simulink model "DKSTDD_Bo_KDXCS_dieu_khien_DC_1c"  (R2019a)
settings: Solver=VariableStepAuto  StartTime=0.0  StopTime=5  RelTol=1e-3
libraries: powerlib x8
settings Model: Creator=Admin  LastModifiedBy=Admin

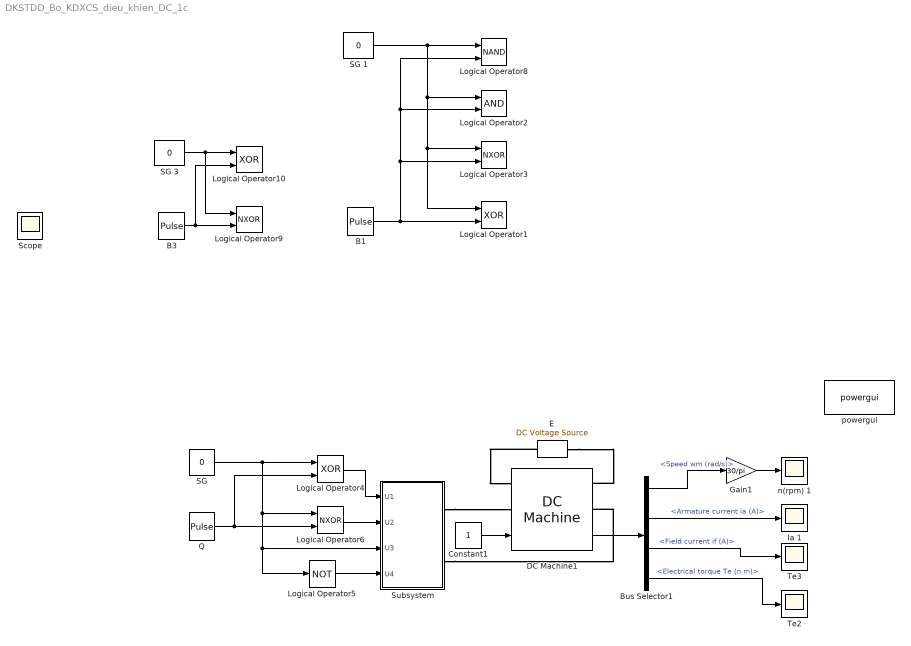
== system DKSTDD_Bo_KDXCS_dieu_khien_DC_1c ==
  B1 : DiscretePulseGenerator  PulseType=Time based  Period=0.002  PulseWidth=20
  B3 : DiscretePulseGenerator  PulseType=Time based  Period=0.002  PulseWidth=20
  Bus Selector1 : BusSelector  OutputSignals=Speed wm (rad/s),Armature current ia (A),Field current if (A),Electrical torque Te (n m)
  Constant1 : Constant
  DC Machine1 : powerlib/Machines/DC Machine  PresetModel=01: 5HP 240V 1750RPM Field:300V  MechanicalLoad=Torque TL  FieldType=Wound  ShowDetailedParameters=on  MeasurementBus=off  RLa=[2.581 0.028]  RLf=[281.3 156]  Laf=0.9483  MachineConstant=Torque constant (N.m/A)  Ke=1.8  Kt=1.8  J=0.02215  Bm=0.002953  Tf=0.5161  w0=1  Ifinit=1  TsPowergui=0  TsBlock=-1
  E : powerlib/Electrical Sources/DC Voltage Source  Amplitude=300  Measurements=None
  Gain1 : Gain  Gain=30/pi
  Ia 1 : Scope
  Logical Operator1 : Logic  Operator=XOR  AllPortsSameDT=off  OutDataTypeStr=boolean
  Logical Operator10 : Logic  Operator=XOR  AllPortsSameDT=off  OutDataTypeStr=boolean
  Logical Operator2 : Logic  AllPortsSameDT=off  OutDataTypeStr=boolean
  Logical Operator3 : Logic  Operator=NXOR  AllPortsSameDT=off  OutDataTypeStr=boolean
  Logical Operator4 : Logic  Operator=XOR  AllPortsSameDT=off  OutDataTypeStr=boolean
  Logical Operator5 : Logic  Operator=NOT  AllPortsSameDT=off  OutDataTypeStr=boolean
  Logical Operator6 : Logic  Operator=NXOR  AllPortsSameDT=off  OutDataTypeStr=boolean
  Logical Operator8 : Logic  Operator=NAND  AllPortsSameDT=off  OutDataTypeStr=boolean
  Logical Operator9 : Logic  Operator=NXOR  AllPortsSameDT=off  OutDataTypeStr=boolean
  Q : DiscretePulseGenerator  PulseType=Time based  Period=0.002  PulseWidth=20
  SG : Constant  Value=0
  SG 1 : Constant  Value=0
  SG 3 : Constant  Value=0
  Scope : Scope  NumInputPorts=4
  Subsystem : Subsystem
  Te2 : Scope
  Te3 : Scope
  n(rpm) 1 : Scope
  powergui : powerlib/powergui  Priority=1  SimulationMode=Continuous  SampleTime=50e-6  frequency=60  Iterations=50  frequencyindice=0  Pbase=100e6  ErrMax=1e-4  UnitsV=kV  UnitsW=MW  buscounter=0  FunctionMessages=off  echomessages=off  EnableUseOfTLC=off  CurrentSourceSwitches=off  DisableSnubberDevices=off  DisableRonSwitches=off  DisableVfSwitches=off  DisplayEquations=off  AutomaticDiscreteSolvers=off  SolverType=Tustin/Backward Euler (TBE)  Interpol=off  ExternalGateDelay=off  methode=off  Ts=100  x0status=blocks  SPID=on  SwTol=0  HookPort=off  NonlinearTolerance=0  nMaxIteration=15  ContinueOnMaxIteration=off  RestoreLinks=warning  ResistiveCurrentMeasurement=off  Frange=[0:2:500]  Ylog=off  Xlog=on  ShowGrid=off  save=off  variable=ZData  structure=0  ZoomFFT=off  StartTime=0.0  cycles=1  DisplayStyle=1  fundamental=60  FreqAxis=off  MaxFrequency=1000  frequencyindicesteady=1  RmsSteady=1  display=off
      settings: SourceProductName=Simscape Electrical
  wires:
  Bus Selector1/1 -> Gain1/1  "<Speed wm (rad/s)>"
  Bus Selector1/4 -> Te2/1  "<Electrical torque Te (n m)>"
  Bus Selector1/2 -> Ia 1/1  "<Armature current ia (A)>"
  Constant1/1 -> DC Machine1/1
  Gain1/1 -> n(rpm) 1/1
  Bus Selector1/3 -> Te3/1  "<Field current if (A)>"
  DC Machine1/1 -> Bus Selector1/1
  Logical Operator4/1 -> Subsystem/1(U1)
  Logical Operator6/1 -> Subsystem/2(U2)
  SG/1 -> Subsystem/3(U3), Logical Operator5/1, Logical Operator6/1, Logical Operator4/1
  Q/1 -> Logical Operator6/2, Logical Operator4/2
  SG 1/1 -> Logical Operator1/1, Logical Operator3/1, Logical Operator2/1, Logical Operator8/1
  B1/1 -> Logical Operator3/2, Logical Operator2/2, Logical Operator8/2, Logical Operator1/2
  SG 3/1 -> Logical Operator9/1, Logical Operator10/1
  B3/1 -> Logical Operator9/2, Logical Operator10/2
  Logical Operator5/1 -> Subsystem/4(U4)
  connections:
  E/LConn1 -- DC Machine1/RConn2
  E/RConn1 -- DC Machine1/LConn2
  Subsystem/RConn1 -- DC Machine1/LConn1
  Subsystem/RConn2 -- DC Machine1/RConn1

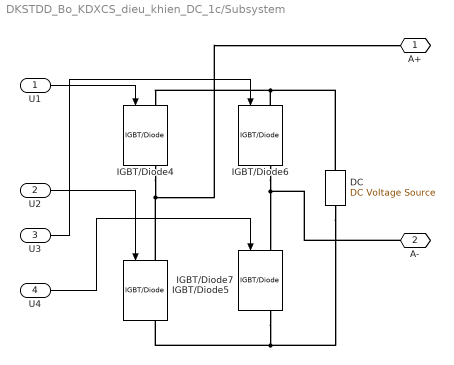
== system DKSTDD_Bo_KDXCS_dieu_khien_DC_1c/Subsystem ==
  U1 : Inport
  U2 : Inport  Port=2
  U3 : Inport  Port=3
  U4 : Inport  Port=4
  DC : powerlib/Electrical Sources/DC Voltage Source  Amplitude=240  Measurements=None
  IGBT/Diode{4..7} (4 alike) : powerlib/Power Electronics/IGBT//Diode  Ron=1e-3  Rs=1e5  Cs=inf  Measurements=on
      settings: SourceProductName=Simscape Electrical
  A+ : PMIOPort  Side=Right
  A- : PMIOPort  Port=2  Side=Right
  wires:
  U1/1 -> IGBT/Diode4/1
  U4/1 -> IGBT/Diode7/1
  U2/1 -> IGBT/Diode5/1
  U3/1 -> IGBT/Diode6/1
  connections:
  IGBT/Diode5/LConn1 -- IGBT/Diode4/RConn1 -- A+/RConn1
  DC/RConn1 -- IGBT/Diode6/LConn1 -- IGBT/Diode4/LConn1
  IGBT/Diode6/RConn1 -- A-/RConn1 -- IGBT/Diode7/LConn1
  DC/LConn1 -- IGBT/Diode7/RConn1 -- IGBT/Diode5/RConn1
